simulink model "psd_regulator_prudu1"  (R2015a)
settings: Solver=ode3  StartTime=0.0  StopTime=0.9  FixedStep=periodaCurrent  RelTol=1e-3
values from neighbouring files (symbols this model uses):
  p1 = ((kiCurrent-kdCurrent)/(kpCurrent+kiCurrent+kdCurrent))    (= 0.0184049079755)    [plot_current_step_with_reg.m]
  p2 = ((kdCurrent)/(kpCurrent+kiCurrent+kdCurrent))    (= 0)    [plot_current_step_with_reg.m]
  periodaCurrent = 0.0015    [plot_current_step_with_reg.m]
  q0 = (kpCurrent+kdCurrent)    (= 2)    [plot_current_step_with_reg.m]
  q1 = (-kpCurrent-2*kdCurrent+kiCurrent)    (= -1.9625)    [plot_current_step_with_reg.m]
  q2 = kdCurrent    (= 0)    [plot_current_step_with_reg.m]
  stepValue = 80    [plot_current_step_with_reg.m]
settings Model: Creator=Juraj  LastModifiedBy=Juraj

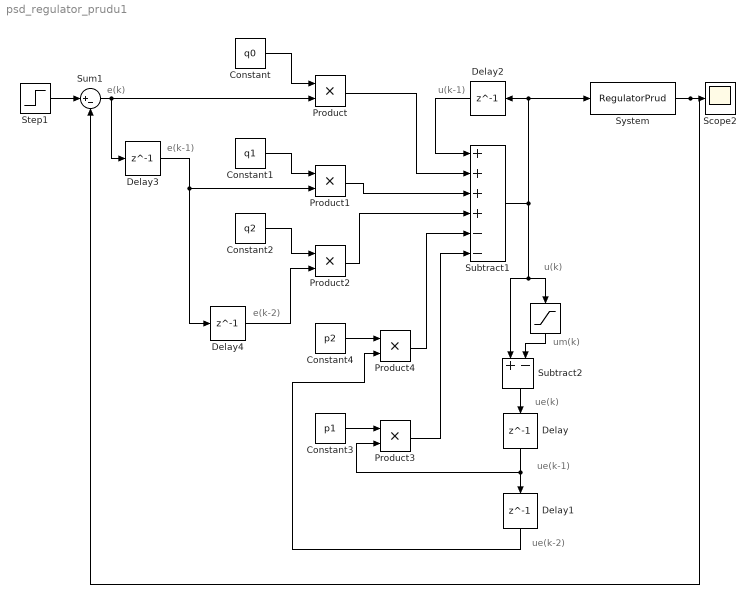
== system psd_regulator_prudu1 ==
  note: e(k-2)
  note: e(k-1)
  note: e(k)
  note: u(k-1)
  note: ue(k-2)
  note: ue(k)
  note: ue(k-1)
  note: u(k)
  note: um(k)
  " " : Saturate  UpperLimit=255  LowerLimit=0
  Constant : Constant  Value=q0
  Constant1 : Constant  Value=q1
  Constant2 : Constant  Value=q2
  Constant3 : Constant  Value=p1
  Constant4 : Constant  Value=p2
  Delay{,1..4} (5 alike) : Delay  DelayLength=1  InitialCondition=0  SampleTime=periodaCurrent
  Product{,1..4} (5 alike) : Product
  Scope2 : Scope
      settings: YMin=48.05  YMax=49.15  SaveName=ScopeData2
  Step1 : Step  Time=0  After=stepValue  SampleTime=0
  Subtract1 : Sum  Inputs=++++--
  Subtract2 : Sum  Inputs=+-
  Sum1 : Sum  Inputs=|+-
  System : M-S-Function  FunctionName=RegulatorPrud
  wires:
  " "/1 -> Subtract2/2
  Delay/1 -> Delay1/1, Product3/2
  Step1/1 -> Sum1/1
  System/1 -> Sum1/2, Scope2/1
  Sum1/1 -> Delay3/1, Product/2
  Delay2/1 -> Subtract1/1
  Constant/1 -> Product/1
  Product/1 -> Subtract1/2
  Delay3/1 -> Delay4/1, Product1/2
  Constant1/1 -> Product1/1
  Product1/1 -> Subtract1/3
  Delay4/1 -> Product2/2
  Constant2/1 -> Product2/1
  Product2/1 -> Subtract1/4
  Constant3/1 -> Product3/1
  Delay1/1 -> Product4/2
  Constant4/1 -> Product4/1
  Subtract1/1 -> Subtract2/1, " "/1, System/1, Delay2/1
  Subtract2/1 -> Delay/1
  Product3/1 -> Subtract1/6
  Product4/1 -> Subtract1/5
